simulink model "controladorP"  (Simulink 7.9)
settings: Solver=ode45  StartTime=0.0  StopTime=5000  MaxStep=0.03  MinStep=0.01  RelTol=1e-3
settings Model: Creator=Daniel  LastModifiedBy=root
settings SolverCC: InitialStep=0.01
settings DebuggingCC: FcnCallInpInsideContextMsg=Use local settings  StrictBusMsg=Warning
settings GRTTargetCC: CombineOutputUpdateFcns=off  GRTInterface=on

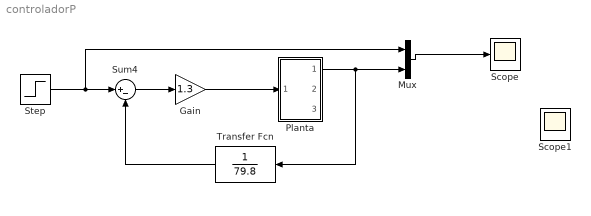
== system controladorP ==
  Gain : Gain  Gain=1.3
  Mux : Mux  Inputs=2
  Planta : Subsystem
  Scope : Scope
      settings: TimeRange=1000  YMin=25  YMax=65
  Scope1 : Scope
  Step : Step  After=30  SampleTime=0.1
  Sum4 : Sum  Inputs=|+-  SampleTime=0.1
  Transfer Fcn : TransferFcn  Denominator=[0 79.8]
  wires:
  Planta/1(Out1) -> Mux/2, Transfer Fcn/1
  Mux/1 -> Scope/1
  Sum4/1 -> Gain/1
  Gain/1 -> Planta/1(In1)
  Step/1 -> Sum4/1, Mux/1
  Transfer Fcn/1 -> Sum4/2

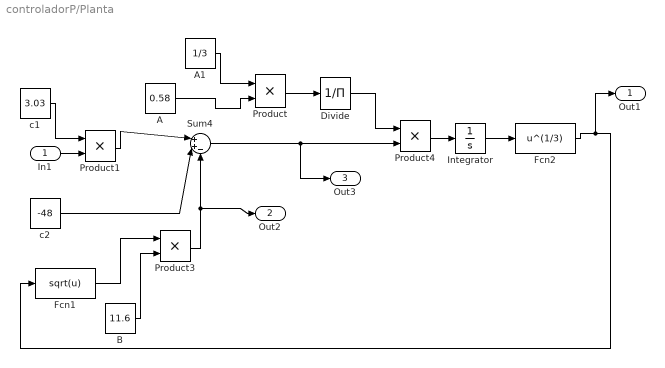
== system controladorP/Planta ==
  In1 : Inport
  A : Constant  Value=0.58
  A1 : Constant  Value=1/3
  B : Constant  Value=11.6
  Divide : Product  Inputs=/
  Fcn1 : Fcn  Expr=sqrt(u)  SampleTime=0.1
  Fcn2 : Fcn  Expr=u^(1/3)  SampleTime=0.1
  Integrator : Integrator  LowerSaturationLimit=0.1
  Product : Product  Inputs=**  RndMeth=Zero
  Product1 : Product  SampleTime=0.1  RndMeth=Zero
  Product3 : Product  SampleTime=0.1  RndMeth=Zero
  Product4 : Product  SampleTime=0.1  RndMeth=Zero
  Sum4 : Sum  Inputs=|++-
  c1 : Constant  Value=3.03
  c2 : Constant  Value=-48
  Out1 : Outport
  Out2 : Outport  Port=2
  Out3 : Outport  Port=3
  wires:
  c1/1 -> Product1/1
  Product1/1 -> Sum4/1
  c2/1 -> Sum4/2
  Fcn1/1 -> Product3/1
  B/1 -> Product3/2
  Product3/1 -> Sum4/3, Out2/1
  Sum4/1 -> Product4/2, Out3/1
  Divide/1 -> Product4/1
  Product/1 -> Divide/1
  Product4/1 -> Integrator/1
  In1/1 -> Product1/2
  A/1 -> Product/2
  A1/1 -> Product/1
  Integrator/1 -> Fcn2/1
  Fcn2/1 -> Fcn1/1, Out1/1
